simulink model "OBSWAM_var"  (Simulink 7.4)
settings: Solver=ode45  StartTime=0.0  StopTime=8  MinStep=0.01  RelTol=1e-3
values from neighbouring files (symbols this model uses):
  Kact = eye(7)    [batchwamobs.m]
  Kd = Kp.^0.5*2    [WAMforcecontrol.m]    (also in batchwamobs.m = 50*eye(7); paralelcontrol2R.m = eye(n)*1000)
  Kp = 25*eye(7)    [batchwamobs.m]    (also in paralelcontrol2R.m = eye(n)*2500)
  wam = robot(L, 'Wam arm', 'Barrett', 'dh params')    [WAM.m]
undefined symbols (not defined in the file or in its folder): Kd1, Kp1, uextgeneratorwam
libraries: roblocks x2
settings Model: Creator=acolome  LastModifiedBy=acolome

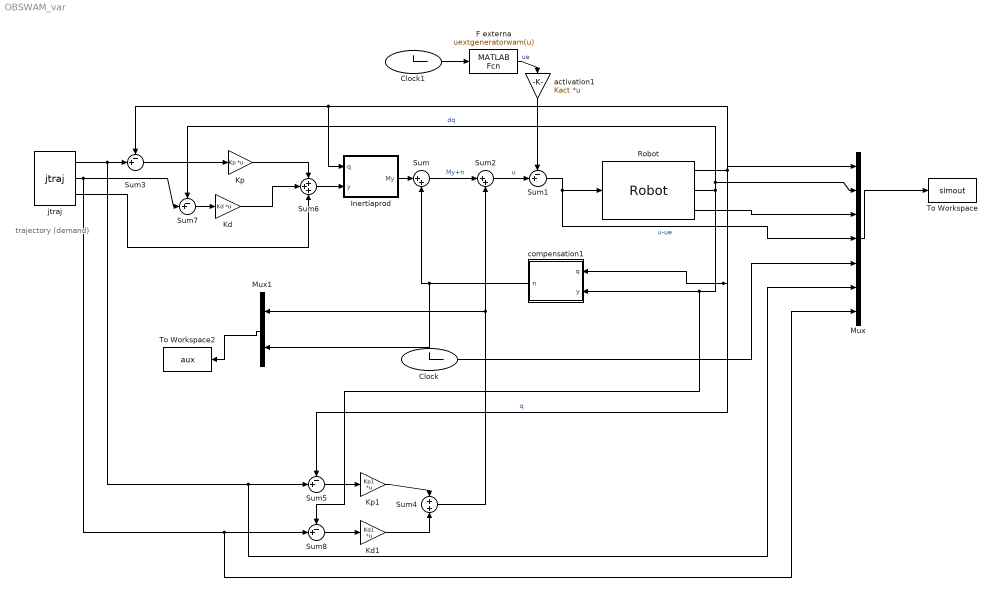
== system OBSWAM_var ==
  note: trajectory
      | (demand)
  Clock : Clock
      settings: Decimation=100
  Clock1 : Clock
      settings: Decimation=100
  F externa : MATLABFcn  MATLABFcn=uextgeneratorwam(u)  OutputDimensions=7
  Inertiaprod : Subsystem  mask{robot=wam, g=[0 0 9.81]}
      mask prompts: robot "Robot Object"; g "Gravity"
      mask init:
      | n=robot.n
      mask Display:
      | port_label('output',1,'M(q)y')
      | 
      | port_label('input', 1, 'q')
      | port_label('input', 2, 'y')
  Kd : Gain  Gain=Kd  Multiplication=Matrix(K*u)  SaturateOnIntegerOverflow=on  OutDataTypeStr=Inherit: Same as input  ParamDataTypeStr=Inherit: Same as input
  Kd1 : Gain  Gain=Kd1  Multiplication=Matrix(K*u)  SaturateOnIntegerOverflow=on  OutDataTypeStr=Inherit: Same as input  ParamDataTypeStr=Inherit: Same as input
  Kp : Gain  Gain=Kp  Multiplication=Matrix(K*u)  SaturateOnIntegerOverflow=on  OutDataTypeStr=Inherit: Same as input  ParamDataTypeStr=Inherit: Same as input
  Kp1 : Gain  Gain=Kp1  Multiplication=Matrix(K*u)  SaturateOnIntegerOverflow=on  OutDataTypeStr=Inherit: Same as input  ParamDataTypeStr=Inherit: Same as input
  Mux : Mux  Inputs=7
  Mux1 : Mux  Inputs=2
  Robot : roblocks/Robot  SystemSampleTime=-1  robot=wam  q0=[0 0 0 0 0 0 0]
  Sum : Sum  Inputs=|++  OutDataType=fixdt(1, 16)  OutScaling=2^0
  Sum1 : Sum  Inputs=-+|  OutDataType=fixdt(1, 16)  OutScaling=2^0
  Sum2 : Sum  Inputs=|++  OutDataType=fixdt(1, 16)  OutScaling=2^0
  Sum{3,5,7..8} (4 alike) : Sum  Inputs=-+|  SaturateOnIntegerOverflow=on  InputSameDT=on  OutDataTypeStr=Inherit: Same as first input
  Sum4 : Sum  OutDataType=fixdt(1, 16)  OutScaling=2^0
  Sum6 : Sum  Inputs=+++  OutDataType=fixdt(1, 16)  OutScaling=2^0
  To Workspace : ToWorkspace  VariableName=simout  SampleTime=-1  SaveFormat=Array
  To Workspace2 : ToWorkspace  VariableName=aux  SampleTime=-1  SaveFormat=Array
  activation1 : Gain  Gain=Kact  Multiplication=Matrix(K*u)  SaturateOnIntegerOverflow=on  OutDataTypeStr=Inherit: Same as input  ParamDataTypeStr=Inherit: Same as input
  compensation1 : Subsystem  mask{robot=wam, g=[0 0 9.81]}
      mask prompts: robot "Robot Object"; g "Gravity"
      mask init:
      | n=robot.n
      mask Display:
      | port_label('output',1,'n(q,dq)')
      | 
      | port_label('input', 1, 'q')
      | port_label('input', 2, 'dq')
  jtraj : roblocks/jtraj  SystemSampleTime=-1  q0=[0 0 0 0 0 0 0]*0  qf=[1 1 1 1 1 1 1]  tmax=8
      link override MATLAB Fcn: MATLABFcn=squeeze(interp1(t,q,u))
      link override MATLAB Fcn1: MATLABFcn=squeeze(interp1(t,qd,u))
      link override MATLAB Fcn2: MATLABFcn=squeeze(interp1(t,qdd,u))
  wires:
  Mux/1 -> To Workspace/1
  jtraj/2 -> Sum7/2, Sum8/2, Mux/7
  Sum7/1 -> Kd/1
  Sum3/1 -> Kp/1
  jtraj/3 -> Sum6/3
  Kd/1 -> Sum6/2
  Kp/1 -> Sum6/1
  jtraj/1 -> Sum3/2, Sum5/2, Mux/6
  Robot/1 -> Sum3/1, Inertiaprod/1(q), Mux/1, compensation1/1(q), Sum5/1  "q"
  Robot/2 -> Sum7/1, Mux/2, compensation1/2(y), Sum8/1  "dq"
  Sum6/1 -> Inertiaprod/2(y)
  Robot/3 -> Mux/3
  Clock/1 -> Mux/5
  compensation1/1(n) -> Sum/2, Mux1/2
  Sum1/1 -> Robot/1, Mux/4  "u-ue"
  Inertiaprod/1(My) -> Sum/1
  Clock1/1 -> F externa/1
  Sum/1 -> Sum2/1  "My+n"
  Sum2/1 -> Sum1/2  "u"
  F externa/1 -> activation1/1  "ue"
  activation1/1 -> Sum1/1
  Mux1/1 -> To Workspace2/1
  Sum5/1 -> Kp1/1
  Sum8/1 -> Kd1/1
  Kp1/1 -> Sum4/1
  Kd1/1 -> Sum4/2
  Sum4/1 -> Sum2/2, Mux1/1

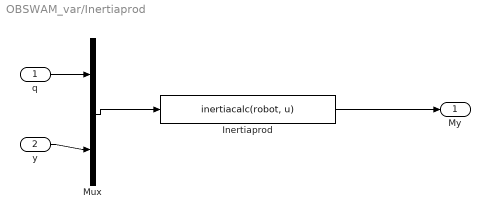
== system OBSWAM_var/Inertiaprod ==
  q : Inport  OutDataType=fixdt(1, 16)  OutScaling=2^0
  y : Inport  Port=2  OutDataType=fixdt(1, 16)  OutScaling=2^0
  Inertiaprod : MATLABFcn  MATLABFcn=inertiacalc(robot, u)  OutputDimensions=n
  Mux : Mux  Inputs=2
  My : Outport  OutDataType=fixdt(1, 16)  OutScaling=2^0
  wires:
  Mux/1 -> Inertiaprod/1
  q/1 -> Mux/1
  Inertiaprod/1 -> My/1
  y/1 -> Mux/2

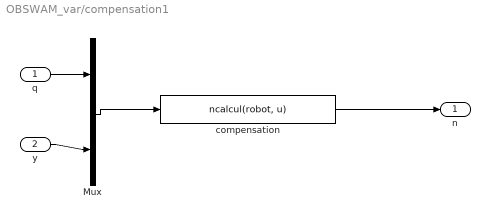
== system OBSWAM_var/compensation1 ==
  q : Inport  OutDataType=fixdt(1, 16)  OutScaling=2^0
  y : Inport  Port=2  OutDataType=fixdt(1, 16)  OutScaling=2^0
  Mux : Mux  Inputs=2
  compensation : MATLABFcn  MATLABFcn=ncalcul(robot, u)  OutputDimensions=n
  n : Outport  OutDataType=fixdt(1, 16)  OutScaling=2^0
  wires:
  Mux/1 -> compensation/1
  q/1 -> Mux/1
  compensation/1 -> n/1
  y/1 -> Mux/2
